simulink model "Assignment1_StateFlow"  (R2017a)
settings: Solver=VariableStepAuto  StartTime=0.0  StopTime=10.0  RelTol=1e-3
undefined symbols (not defined in the file): D2, PTB9
libraries: frdmk64flib x1
settings Model: Creator=samacl  LastModifiedBy=samacl

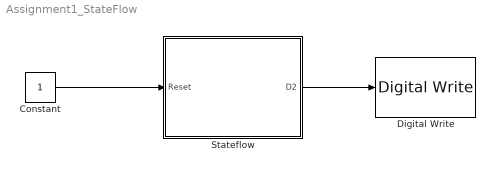
== system Assignment1_StateFlow ==
  Constant : Constant
  Digital Write : frdmk64flib/Digital Write  Whichpin=PTB9 (D2)
      settings: SourceProductName=Simulink Coder Support Package for NXP FRDM-K64F Board
  Stateflow : Stateflow chart  TreatAsAtomicUnit=on
  wires:
  Stateflow/1(D2) -> Digital Write/1
  Constant/1 -> Stateflow/1(Reset)

== stateflow chart Assignment1_StateFlow/Stateflow ==
  note: Wait for VRP
  state Sense_v
    entry: sense_ventricle()
  state Pulse_v
    entry: pulse_ventricle()
  state Set_v
    entry: set_ventricle()
  note: Wait for VRP
  state Load
    entry: load_data(Reset)
  state Pulse_a
    entry: pulse_atrium()
  note: Wait for ARP
  state Set_a
    entry: set_atrium()
  note: Wait for ARP
  state Sense_a
    entry: sense_atrium()
  Sense_v -> Load [order 1]
  Sense_v -> Pulse_v [order 2]
  Set_v -> Sense_v [order 1]
  Pulse_v -> Load
  Set_v -> Pulse_v [order 2]
  Load -> Set_v [order 2]
  Pulse_a -> Set_v [order 2]
  Pulse_a -> Load [order 1]
  (default) -> Load
  Set_a -> Pulse_a [order 2]
  Sense_a -> Pulse_a [order 2]
  Sense_a -> Load [order 1]
  Load -> Set_a [order 1]
  Set_a -> Sense_a [order 1]
  data: x function_input; Reset input; D2 output
  function load_data(x):
    | % Load all parameters from DCM
    | % Load mode
    | % Checks Magnet
    | % Checks if Reset button was pressed by the doctor
    | function load_data(x)
    |     if(x)
    |         
    |     end
    | end
  function set_ventricle:
    | % million switch statements
    | % charge capacitor
    | % 
    | function set_ventricle()
    | 
    | end
  function set_atrium:
    | function set_atrium()
    | 
    | end
  function sense_ventricle:
    | % check if the heart pulsed
    | % if the heart pulsed go to load
    | % else pulse
    | function sense_ventricle()
    | 
    | end
  function sense_atrium:
    | % check if the heart pulsed
    | % if the heart pulsed go to load
    | % else pulse
    | function sense_atrium()
    | 
    | end
  function pulse_ventricle:
    | % Discharge capacitor
    | % Pulse between LRL and URL
    | % at the end - wait for the 
    | function pulse_ventricle()
    | 
    | end
  function pulse_atrium:
    | function pulse_atrium()
    | 
    | end
